simulink model "boat_sim_ss_bruce"  (R2018b)
settings: Solver=VariableStepAuto  StartTime=0.0  StopTime=100  RelTol=1e-3
values from neighbouring files (symbols this model uses):
  state_eq = ss(eval(real(linearized_A)), eval(real(linearized_B)), C, D)    [ss_linearization.m]
undefined symbols (not defined in the file or in its folder): K
settings Model: Creator=brucecui  LastModifiedBy=brucecui

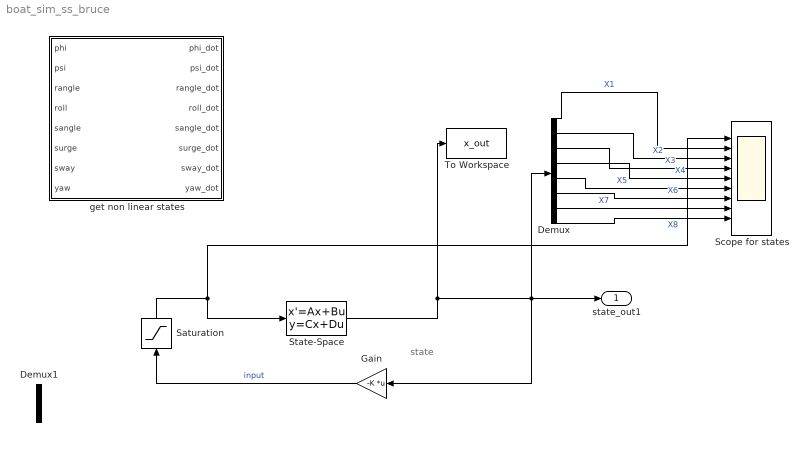
== system boat_sim_ss_bruce ==
  note: state
  Demux : Demux  Outputs=8
  Demux1 : Demux  Outputs=2
  Gain : Gain  Gain=-K  Multiplication=Matrix(K*u)
  Saturation : Saturate  UpperLimit=pi/6  LowerLimit=-pi/6
  Scope for states : Scope  NumInputPorts=9
  State-Space : StateSpace  A=state_eq.a  B=state_eq.b  C=eye(size(state_eq.a))  D=zeros(8,2)  InitialCondition=[1,1,0,0,0,0,0,0]  ContinuousStateAttributes='Velocity'
  To Workspace : ToWorkspace  VariableName=x_out  SampleTime=-1
  "get non linear states " : MATLAB Function  TreatAsAtomicUnit=on
  state_out1 : Outport
  wires:
  Demux/2 -> Scope for states/3  "X2"
  State-Space/1 -> To Workspace/1, Demux/1, Gain/1, state_out1/1
  Demux/1 -> Scope for states/2  "X1"
  Demux/3 -> Scope for states/4  "X3"
  Demux/4 -> Scope for states/5  "X4"
  Gain/1 -> Saturation/1  "input"
  Demux/5 -> Scope for states/6  "X5"
  Demux/6 -> Scope for states/7  "X6"
  Demux/7 -> Scope for states/8  "X7"
  Demux/8 -> Scope for states/9  "X8"
  Saturation/1 -> Scope for states/1, State-Space/1

== matlab function boat_sim_ss_bruce/get non linear states  ==
  data: phi input; phi_dot output; psi input; rangle input; roll input; sangle input; surge input; sway input; yaw input; psi_dot output; rangle_dot output; roll_dot output; sangle_dot output; surge_dot output; sway_dot output; yaw_dot output
function [phi_dot, psi_dot, rangle_dot, roll_dot, sangle_dot, surge_dot, sway_dot, yaw_dot]= fcn(phi, psi, rangle, roll, sangle, surge, sway, yaw)

    [phi_dot, psi_dot, rangle_dot, roll_dot, sangle_dot, surge_dot, sway_dot, yaw_dot]=get_non_linear_states(phi, psi, rangle, roll, sangle, surge, sway, yaw);

end
